simulink model "matlab_mixed_cosim"  (Simulink 7.0)
settings: Solver=FixedStepDiscrete  SolverMode=SingleTasking  StartTime=0.0  StopTime=370  RelTol=1e-3
undefined symbols (not defined in the file or in its folder): ieee_nowarn, image, port_label
libraries: aldec_ahdl x7
settings Model: Creator=arekg  LastModifiedBy=arekg
settings DataIOCC: SignalLoggingName=sigsOut
settings OptimizationCC: InlineInvariantSignals=on
settings DebuggingCC: SaveWithParameterizedLinksMsg=none  SignalResolutionControl=TryResolveAllWithWarning  SolverPrmCheckMsg=none  MultiTaskDSMMsg=warning  MultiTaskCondExecSysMsg=none
settings HardwareCC: TargetUnknown=on
settings RTWCC: IncludeERTFirstTime=on
settings GRTTargetCC: TargetFcnLib=ansi_tfl_tmw.mat  ModelReferenceCompliant=off  MatFileLogging=off

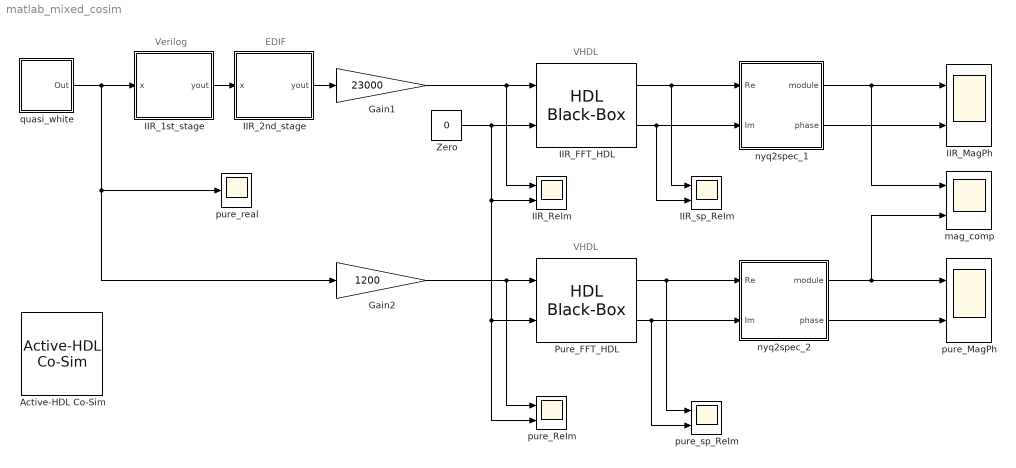
== system matlab_mixed_cosim ==
  note: Verilog
  note: EDIF
  note: VHDL
  note: VHDL
  Active-HDL Co-Sim : aldec_ahdl/Active-HDL Co-Sim  Tag=Active-HDL_Co-Sim_close  Priority=1  hdl_period=0.5  hdl_tscale=sec  sys_period=[1, 0]  sys_tscale=As In Simulator  vsim_cmd=-ieee_nowarn  wav_fn=matlab_mixed_cosim  wav_settings=[0,0,0,0,0,0,0,0]  dbg=off  auto_start=off  gen_tb=[0,0,0]  batch_sim=off  tb_fn=mlab_post_tb.log  metavalue_map=[0,0]  sim_resolution=[1,0,0]  active_page=4  aws_en=off  ahdl_en=off  blk_ver=9.3.RTM  macro_en=[1,0,1]  macro_path=prepare_project.do  mfun_text=check_mfiles
  Gain1 : Gain  Gain=23000  ParameterDataType=sfix(16)  ParameterScaling=2^0  OutDataType=sfix(16)  OutScaling=2^0  SaturateOnIntegerOverflow=on
  Gain2 : Gain  Gain=1200  ParameterDataType=sfix(16)  ParameterScaling=2^0  OutDataType=sfix(16)  OutScaling=2^0  SaturateOnIntegerOverflow=on
  IIR_1st_stage : Subsystem
  IIR_2nd_stage : Subsystem
  IIR_FFT_HDL : aldec_ahdl/HDL Black-Box  Priority=1  module_m=top_fft  ports_cfg={ce,4,1,0,0,1,8,0,0,1,0,0}{clk,3,1,0,0,1,8,0,0,1,0,0}{inv,5,1,0,0,1,8,0,0,1,0,0}{rst,5,1,0,0,1,8,0,0,1,0,0}{start,5,1,0,0,1,8,0,0,1,0,0}{Iin,0,-1,0,0,Inherited,0,0,0,0,0,0}{Qin,0,-1,0,0,Inherited,0,0,0,0,0,0}{Iout,1,-1,0,0,clk,0,0,0,0,0,0}{Qout,1,-1,0,0,clk,0,0,0,0,0,0}  params={WIDTH,16,NATURAL}{POINT,64,NATURAL}{STAGE,3,NATURAL}  clocks={1,2,0,0.5000,0}  ces={0,1,1,0,1}  stims={3,1 0s 0 7s}{4,0 0s 1 8s 0 10s}{2,0}  hdl_src=c:\My_Designs\Samples_73\simulink_mixed_example\fft\src\cfft\address.vhd;c:\My_Designs\Samples_73\simulink_mixed_example\fft\src\cfft\blockdram.vhd;c:\My_Designs\Samples_73\simulink_mixed_example\fft\src\cfft\div4limit.vhd;c:\My_Designs\Samples_73\simulink_mixed_example\fft\src\cfft\cfft4.vhd;c:\My_Designs\Samples_73\simulink_mixed_example\fft\src\cfft\rofactor.vhd;c:\My_Designs\Samples_73\simulink_mixed_example\fft\src\cfft\p2r_cordic.vhd;c:\My_Designs\Samples_73\simulink_mixed_example\fft\src\cfft\sc_corproc.vhd;c:\My_Designs\Samples_73\simulink_mixed_example\fft\src\cfft\mulfactor.vhd;c:\My_Designs\Samples_73\simulink_mixed_example\fft\src\cfft\cfft.vhd;c:\My_Designs\Samples_73\simulink_mixed_example\fft\src\ram\ram.vhd;c:\My_Designs\Samples_73\simulink_mixed_example\fft\compile\control.vhd;c:\My_Designs\Samples_73\simulink_mixed_example\fft\compile\top_fft.vhd  block_mask=image(imread('HDLBlackBox.jpg'),'center'); disp('top_fft');port_label('input', 1, 'Iin');port_label('input', 2, 'Qin');port_label('output', 1, 'Iout');port_label('output', 2, 'Qout');  config=[2,2]  inp=[2, 0, abs(16-1 - 0) + 1, 0, 0, 0, 0, 0, abs(16-1 - 0) + 1, 0, 0, 0, 0]  out=[2, 0, abs(16+1 - 0) + 1, 0, 0, 0, 0, 0, abs(16+1 - 0) + 1, 0, 0, 0, 0]  sampling=[1,-1,-1,2,2]  active_page={0}{80,0,35,1,65,2,70,3,70,4,60,5,60,6,50,7,35,8,35,9,119,10}{103,0,55,1,70,2,75,3,75,4,45,5,45,6,45,7,165,8,0,0,0,0}{165,0,130,1,190,2,190,3,0,0,0,0,0,0,0,0,0,0,0,0,0,0}{81,0,60,1,60,2,70,3,60,4,0,0,0,0,0,0,0,0,0,0,0,0}{83,0,70,1,80,2,50,3,50,4,0,0,0,0,0,0,0,0,0,0,0,0}{125,0,330,1,220,2,0,0,0,0,0,0,0,0,0,0,0,0,0,0,0,0}{95,0,95,1,70,2,50,3,80,4,35,5,35,6,65,7,150,8,0,0,0,0}{735,436}  param_val={16,-1,64,-1,3,-1}  clk_val=[2,0,0.5000]  ce_val=[1,0]  blk_ver=9.3.RTM  blk_conf=0  user_conv=0
  IIR_MagPh : Scope  NumInputPorts=2
      settings: YMin=0~-2  YMax=11500~3.25
  IIR_ReIm : Scope  NumInputPorts=2
      settings: YMin=-25000~-1  YMax=25000~1  SaveName=ScopeData19
  IIR_sp_ReIm : Scope  NumInputPorts=2
      settings: YMin=-35000~-35000  YMax=35000~35000  SaveName=ScopeData5
  Pure_FFT_HDL : aldec_ahdl/HDL Black-Box  Priority=1  module_m=top_fft  ports_cfg={ce,4,1,0,0,1,8,0,0,1,0,0}{clk,3,1,0,0,1,8,0,0,1,0,0}{inv,5,1,0,0,1,8,0,0,1,0,0}{rst,5,1,0,0,1,8,0,0,1,0,0}{start,5,1,0,0,1,8,0,0,1,0,0}{Iin,0,-1,0,0,Inherited,0,0,0,0,0,0}{Qin,0,-1,0,0,Inherited,0,0,0,0,0,0}{Iout,1,-1,0,0,clk,0,0,0,0,0,0}{Qout,1,-1,0,0,clk,0,0,0,0,0,0}  params={WIDTH,16,NATURAL}{POINT,64,NATURAL}{STAGE,3,NATURAL}  clocks={1,2,0,0.5000,0}  ces={0,1,1,0,1}  stims={3,1 0s 0 7s}{4,0 0s 1 8s 0 10s}{2,0}  hdl_src=c:\My_Designs\Samples_73\simulink_mixed_example\fft\src\cfft\address.vhd;c:\My_Designs\Samples_73\simulink_mixed_example\fft\src\cfft\blockdram.vhd;c:\My_Designs\Samples_73\simulink_mixed_example\fft\src\cfft\div4limit.vhd;c:\My_Designs\Samples_73\simulink_mixed_example\fft\src\cfft\cfft4.vhd;c:\My_Designs\Samples_73\simulink_mixed_example\fft\src\cfft\rofactor.vhd;c:\My_Designs\Samples_73\simulink_mixed_example\fft\src\cfft\p2r_cordic.vhd;c:\My_Designs\Samples_73\simulink_mixed_example\fft\src\cfft\sc_corproc.vhd;c:\My_Designs\Samples_73\simulink_mixed_example\fft\src\cfft\mulfactor.vhd;c:\My_Designs\Samples_73\simulink_mixed_example\fft\src\cfft\cfft.vhd;c:\My_Designs\Samples_73\simulink_mixed_example\fft\src\ram\ram.vhd;c:\My_Designs\Samples_73\simulink_mixed_example\fft\compile\control.vhd;c:\My_Designs\Samples_73\simulink_mixed_example\fft\compile\top_fft.vhd  block_mask=image(imread('HDLBlackBox.jpg'),'center'); disp('top_fft');port_label('input', 1, 'Iin');port_label('input', 2, 'Qin');port_label('output', 1, 'Iout');port_label('output', 2, 'Qout');  config=[2,2]  inp=[2, 0, abs(16-1 - 0) + 1, 0, 0, 0, 0, 0, abs(16-1 - 0) + 1, 0, 0, 0, 0]  out=[2, 0, abs(16+1 - 0) + 1, 0, 0, 0, 0, 0, abs(16+1 - 0) + 1, 0, 0, 0, 0]  sampling=[1,-1,-1,2,2]  active_page={0}{80,0,35,1,65,2,70,3,70,4,60,5,60,6,50,7,35,8,35,9,119,10}{103,0,55,1,70,2,75,3,75,4,45,5,45,6,45,7,165,8,0,0,0,0}{165,0,130,1,190,2,190,3,0,0,0,0,0,0,0,0,0,0,0,0,0,0}{81,0,60,1,60,2,70,3,60,4,0,0,0,0,0,0,0,0,0,0,0,0}{83,0,70,1,80,2,50,3,50,4,0,0,0,0,0,0,0,0,0,0,0,0}{125,0,330,1,220,2,0,0,0,0,0,0,0,0,0,0,0,0,0,0,0,0}{95,0,95,1,70,2,50,3,80,4,35,5,35,6,65,7,150,8,0,0,0,0}{735,436}  param_val={16,-1,64,-1,3,-1}  clk_val=[2,0,0.5000]  ce_val=[1,0]  blk_ver=9.3.RTM  blk_conf=0  user_conv=0
  Zero : Constant  Value=0  OutDataTypeMode=double  OutDataType=sfix(16)  OutScaling=2^0
  mag_comp : Scope  NumInputPorts=2
      settings: TimeRange=370  YMin=0~0  YMax=12000~7000
  nyq2spec_1 : Subsystem
  nyq2spec_2 : Subsystem
  pure_MagPh : Scope  NumInputPorts=2
      settings: TimeRange=370  YMin=-3.5~-5  YMax=3.5~5  SaveName=ScopeData24
  pure_ReIm : Scope  NumInputPorts=2
      settings: YMin=-1200~-1  YMax=1200~1  SaveName=ScopeData21
  pure_real : Scope
      settings: YMin=-450  YMax=450  SaveName=ScopeData13
  pure_sp_ReIm : Scope  NumInputPorts=2
      settings: YMin=-1~-5  YMax=1~5  SaveName=ScopeData20
  quasi_white : Subsystem
  wires:
  IIR_FFT_HDL/1 -> IIR_sp_ReIm/1, nyq2spec_1/1(Re)
  IIR_FFT_HDL/2 -> IIR_sp_ReIm/2, nyq2spec_1/2(Im)
  nyq2spec_1/1(module) -> IIR_MagPh/1, mag_comp/1
  nyq2spec_1/2(phase) -> IIR_MagPh/2
  Zero/1 -> IIR_FFT_HDL/2, IIR_ReIm/2, pure_ReIm/2, Pure_FFT_HDL/2
  quasi_white/1(Out) -> pure_real/1, IIR_1st_stage/1(x), Gain2/1
  nyq2spec_2/1(module) -> pure_MagPh/1, mag_comp/2
  Gain1/1 -> IIR_ReIm/1, IIR_FFT_HDL/1
  IIR_1st_stage/1(yout) -> IIR_2nd_stage/1(x)
  Pure_FFT_HDL/1 -> nyq2spec_2/1(Re), pure_sp_ReIm/1
  Gain2/1 -> pure_ReIm/1, Pure_FFT_HDL/1
  Pure_FFT_HDL/2 -> nyq2spec_2/2(Im), pure_sp_ReIm/2
  nyq2spec_2/2(phase) -> pure_MagPh/2
  IIR_2nd_stage/1(yout) -> Gain1/1

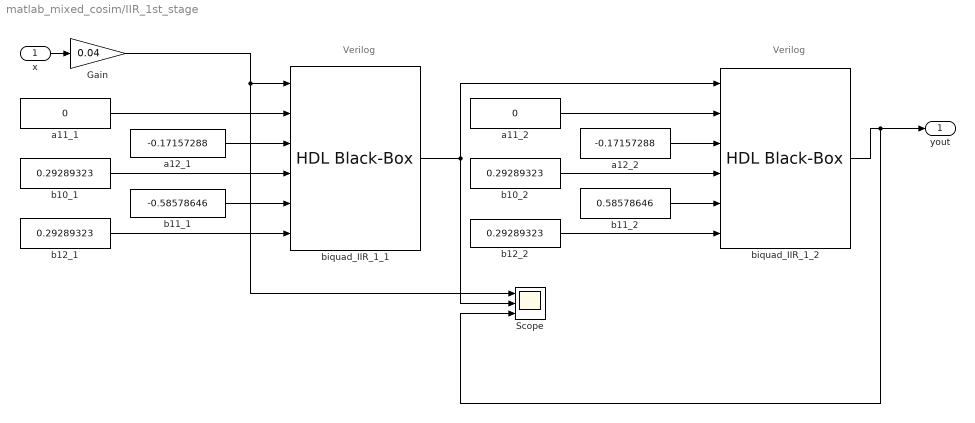
== system matlab_mixed_cosim/IIR_1st_stage ==
  note: Verilog
  note: Verilog
  x : Inport  OutDataType=sfix(16)  OutScaling=2^0
  Gain : Gain  Gain=0.04  ParameterDataType=sfix(16)  ParameterScaling=2^0  OutDataType=sfix(16)  OutScaling=2^0  SaturateOnIntegerOverflow=on
  Scope : Scope  NumInputPorts=3
      settings: YMin=-0.025~-0.025~-0.02  YMax=0.025~0.03~0.03  SaveName=ScopeData3
  a11_1 : Constant  Value=0  OutDataType=sfix(16)  OutScaling=2^0
  a11_2 : Constant  Value=0  OutDataType=sfix(16)  OutScaling=2^0
  a12_1 : Constant  Value=-0.17157288  OutDataType=sfix(16)  OutScaling=2^0
  a12_2 : Constant  Value=-0.17157288  OutDataType=sfix(16)  OutScaling=2^0
  b10_1 : Constant  Value=0.29289323  OutDataType=sfix(16)  OutScaling=2^0
  b10_2 : Constant  Value=0.29289323  OutDataType=sfix(16)  OutScaling=2^0
  b11_1 : Constant  Value=-0.58578646  OutDataType=sfix(16)  OutScaling=2^0
  b11_2 : Constant  Value=0.58578646  OutDataType=sfix(16)  OutScaling=2^0
  b12_1 : Constant  Value=0.29289323  OutDataType=sfix(16)  OutScaling=2^0
  b12_2 : Constant  Value=0.29289323  OutDataType=sfix(16)  OutScaling=2^0
  biquad_IIR_1_1 : aldec_ahdl/HDL Black-Box  Priority=1  module_m=biquad  ports_cfg={clk,3,1,0,0,1,8,0,0,1,0,0}{nreset,5,1,0,0,1,8,0,0,1,0,0}{x,0,16,0,15,Inherited,0,0,0,0,0,0}{ce,4,1,0,0,1,8,0,0,1,0,0}{valid,5,1,0,0,1,8,0,0,1,0,0}{a11,0,8,0,7,Inherited,0,0,0,0,0,0}{a12,0,8,0,7,Inherited,0,0,0,0,0,0}{b10,0,8,0,7,Inherited,0,0,0,0,0,0}{b11,0,8,0,7,Inherited,0,0,0,0,0,0}{b12,0,8,0,7,Inherited,0,0,0,0,0,0}{yout,1,16,0,15,clk,0,0,0,0,0,0}  params={DATAWIDTH,16,}{COEFWIDTH,8,}{ACCUM,2,}  clocks={0,2,0,0.5000,0}  ces={3,0,1,0,1}  stims={4,0 0s 1 2s}{1,0 0s 1 2s}  hdl_src=c:\My_Designs\Samples_73\simulink_mixed_example\biquad_iir\src\multa.v;c:\My_Designs\Samples_73\simulink_mixed_example\biquad_iir\src\multb.v;c:\My_Designs\Samples_73\simulink_mixed_example\biquad_iir\src\biquad.v  block_mask=image(imread('HDLBlackBox.jpg'),'center'); disp('biquad');port_label('input', 1, 'x');port_label('input', 2, 'a11');port_label('input', 3, 'a12');port_label('input', 4, 'b10');port_label('input', 5, 'b11');port_label('input', 6, 'b12');port_label('output', 1, 'yout');  config=[6,1]  inp=[6, 0, 16, 15, 0, 0, 0, 0, 8, 7, 0, 0, 0, 0, 8, 7, 0, 0, 0, 0, 8, 7, 0, 0, 0, 0, 8, 7, 0, 0, 0, 0, 8, 7, 0, 0, 0]  out=[1, 0, 16, 15, 0, 0, 0]  sampling=[1,-1,-1,-1,-1,-1,-1,2]  active_page={0}{80,0,35,1,65,2,70,3,70,4,60,5,60,6,50,7,35,8,35,9,119,10}{103,0,55,1,70,2,75,3,75,4,45,5,45,6,45,7,165,8,0,0,0,0}{165,0,130,1,190,2,190,3,0,0,0,0,0,0,0,0,0,0,0,0,0,0}{81,0,60,1,60,2,70,3,60,4,0,0,0,0,0,0,0,0,0,0,0,0}{83,0,70,1,80,2,50,3,50,4,0,0,0,0,0,0,0,0,0,0,0,0}{125,0,330,1,220,2,0,0,0,0,0,0,0,0,0,0,0,0,0,0,0,0}{95,0,95,1,70,2,50,3,80,4,35,5,35,6,65,7,150,8,0,0,0,0}{735,436}  param_val={16,-1,8,-1,2,-1}  clk_val=[2,0,0.5000]  ce_val=[1,0]  blk_ver=9.3.RTM  blk_conf=0  user_conv=0
  biquad_IIR_1_2 : aldec_ahdl/HDL Black-Box  Priority=1  module_m=biquad  ports_cfg={clk,3,1,0,0,1,8,0,0,1,0,0}{nreset,5,1,0,0,1,8,0,0,1,0,0}{x,0,16,0,15,Inherited,0,0,0,0,0,0}{ce,4,1,0,0,1,8,0,0,1,0,0}{valid,5,1,0,0,1,8,0,0,1,0,0}{a11,0,8,0,7,Inherited,0,0,0,0,0,0}{a12,0,8,0,7,Inherited,0,0,0,0,0,0}{b10,0,8,0,7,Inherited,0,0,0,0,0,0}{b11,0,8,0,7,Inherited,0,0,0,0,0,0}{b12,0,8,0,7,Inherited,0,0,0,0,0,0}{yout,1,16,0,15,clk,0,0,0,0,0,0}  params={DATAWIDTH,16,}{COEFWIDTH,8,}{ACCUM,2,}  clocks={0,2,0,0.5000,0}  ces={3,0,1,0,1}  stims={4,0 0s 1 2s}{1,0 0s 1 2s}  hdl_src=c:\My_Designs\Samples_73\simulink_mixed_example\biquad_iir\src\multa.v;c:\My_Designs\Samples_73\simulink_mixed_example\biquad_iir\src\multb.v;c:\My_Designs\Samples_73\simulink_mixed_example\biquad_iir\src\biquad.v  block_mask=image(imread('HDLBlackBox.jpg'),'center'); disp('biquad');port_label('input', 1, 'x');port_label('input', 2, 'a11');port_label('input', 3, 'a12');port_label('input', 4, 'b10');port_label('input', 5, 'b11');port_label('input', 6, 'b12');port_label('output', 1, 'yout');  config=[6,1]  inp=[6, 0, 16, 15, 0, 0, 0, 0, 8, 7, 0, 0, 0, 0, 8, 7, 0, 0, 0, 0, 8, 7, 0, 0, 0, 0, 8, 7, 0, 0, 0, 0, 8, 7, 0, 0, 0]  out=[1, 0, 16, 15, 0, 0, 0]  sampling=[1,-1,-1,-1,-1,-1,-1,2]  active_page={0}{80,0,35,1,65,2,70,3,70,4,60,5,60,6,50,7,35,8,35,9,119,10}{103,0,55,1,70,2,75,3,75,4,45,5,45,6,45,7,165,8,0,0,0,0}{165,0,130,1,190,2,190,3,0,0,0,0,0,0,0,0,0,0,0,0,0,0}{81,0,60,1,60,2,70,3,60,4,0,0,0,0,0,0,0,0,0,0,0,0}{83,0,70,1,80,2,50,3,50,4,0,0,0,0,0,0,0,0,0,0,0,0}{125,0,330,1,220,2,0,0,0,0,0,0,0,0,0,0,0,0,0,0,0,0}{95,0,95,1,70,2,50,3,80,4,35,5,35,6,65,7,150,8,0,0,0,0}{735,436}  param_val={16,-1,8,-1,2,-1}  clk_val=[2,0,0.5000]  ce_val=[1,0]  blk_ver=9.3.RTM  blk_conf=0  user_conv=0
  yout : Outport  OutDataType=sfix(16)  OutScaling=2^0
  wires:
  x/1 -> Gain/1
  biquad_IIR_1_1/1 -> biquad_IIR_1_2/1, Scope/2
  Gain/1 -> biquad_IIR_1_1/1, Scope/1
  biquad_IIR_1_2/1 -> yout/1, Scope/3
  b10_1/1 -> biquad_IIR_1_1/4
  a12_1/1 -> biquad_IIR_1_1/3
  a11_1/1 -> biquad_IIR_1_1/2
  b12_2/1 -> biquad_IIR_1_2/6
  b10_2/1 -> biquad_IIR_1_2/4
  a12_2/1 -> biquad_IIR_1_2/3
  a11_2/1 -> biquad_IIR_1_2/2
  b11_2/1 -> biquad_IIR_1_2/5
  b12_1/1 -> biquad_IIR_1_1/6
  b11_1/1 -> biquad_IIR_1_1/5

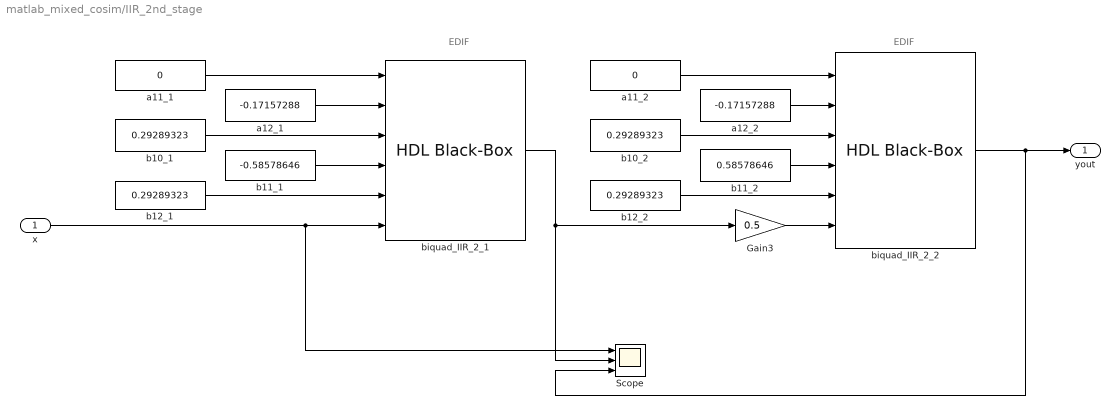
== system matlab_mixed_cosim/IIR_2nd_stage ==
  note: EDIF
  note: EDIF
  x : Inport  OutDataType=sfix(16)  OutScaling=2^0
  Gain3 : Gain  Gain=0.5  ParameterDataType=sfix(16)  ParameterScaling=2^0  OutDataType=sfix(16)  OutScaling=2^0  SaturateOnIntegerOverflow=on
  Scope : Scope  NumInputPorts=3
      settings: YMin=-0.025~-0.025~-0.02  YMax=0.025~0.03~0.03  SaveName=ScopeData4
  a11_1 : Constant  Value=0  OutDataType=sfix(16)  OutScaling=2^0
  a11_2 : Constant  Value=0  OutDataType=sfix(16)  OutScaling=2^0
  a12_1 : Constant  Value=-0.17157288  OutDataType=sfix(16)  OutScaling=2^0
  a12_2 : Constant  Value=-0.17157288  OutDataType=sfix(16)  OutScaling=2^0
  b10_1 : Constant  Value=0.29289323  OutDataType=sfix(16)  OutScaling=2^0
  b10_2 : Constant  Value=0.29289323  OutDataType=sfix(16)  OutScaling=2^0
  b11_1 : Constant  Value=-0.58578646  OutDataType=sfix(16)  OutScaling=2^0
  b11_2 : Constant  Value=0.58578646  OutDataType=sfix(16)  OutScaling=2^0
  b12_1 : Constant  Value=0.29289323  OutDataType=sfix(16)  OutScaling=2^0
  b12_2 : Constant  Value=0.29289323  OutDataType=sfix(16)  OutScaling=2^0
  biquad_IIR_2_1 : aldec_ahdl/HDL Black-Box  Priority=1  module_m=biquad_post_synth  ports_cfg={a11,0,8,0,7,Inherited,0,0,0,0,0,0}{a12,0,8,0,7,Inherited,0,0,0,0,0,0}{b10,0,8,0,7,Inherited,0,0,0,0,0,0}{b11,0,8,0,7,Inherited,0,0,0,0,0,0}{b12,0,8,0,7,Inherited,0,0,0,0,0,0}{x,0,16,0,15,Inherited,0,0,0,0,0,0}{ce,4,1,0,0,1,8,0,0,1,0,0}{clk,3,1,0,0,1,8,0,0,1,0,0}{nreset,5,1,0,0,1,8,0,0,1,0,0}{valid,5,1,0,0,1,8,0,0,1,0,0}{yout,1,16,0,15,clk,0,0,0,0,0,0}  clocks={7,2,0,0.5000,0}  ces={6,7,1,0,1}  stims={8,0 0s 1 2s}{9,0 0s 1 2s}  hdl_src=C:\Program Files\Aldec\Active-HDL 7.2\Vlib\VIRTEX\src\virtex.vhd;C:\Program Files\Aldec\Active-HDL 7.2\Vlib\unisim\src\unisim_vital.vhd;c:\My_Designs\Samples_73\simulink_mixed_example\biquad_iir\src\post-synthesis\biquad_post_synth.edf  block_mask=image(imread('HDLBlackBox.jpg'),'center'); disp('biquad_post_synth');port_label('input', 1, 'a11');port_label('input', 2, 'a12');port_label('input', 3, 'b10');port_label('input', 4, 'b11');port_label('input', 5, 'b12');port_label('input', 6, 'x');port_label('output', 1, 'yout');  config=[6,1]  inp=[6, 0, 8, 7, 0, 0, 0, 0, 8, 7, 0, 0, 0, 0, 8, 7, 0, 0, 0, 0, 8, 7, 0, 0, 0, 0, 8, 7, 0, 0, 0, 0, 16, 15, 0, 0, 0]  out=[1, 0, 16, 15, 0, 0, 0]  sampling=[1,-1,-1,-1,-1,-1,-1,2]  active_page={0}{80,0,35,1,65,2,70,3,70,4,60,5,60,6,50,7,35,8,35,9,119,10}{103,0,55,1,70,2,75,3,75,4,45,5,45,6,45,7,165,8,0,0,0,0}{165,0,130,1,190,2,190,3,0,0,0,0,0,0,0,0,0,0,0,0,0,0}{81,0,60,1,60,2,70,3,60,4,0,0,0,0,0,0,0,0,0,0,0,0}{83,0,70,1,80,2,50,3,50,4,0,0,0,0,0,0,0,0,0,0,0,0}{125,0,330,1,220,2,0,0,0,0,0,0,0,0,0,0,0,0,0,0,0,0}{95,0,95,1,70,2,50,3,80,4,35,5,35,6,65,7,150,8,0,0,0,0}{735,436}  param_val=0  clk_val=[2,0,0.5000]  ce_val=[1,0]  blk_ver=9.3.RTM  blk_conf=0  user_conv=0
  biquad_IIR_2_2 : aldec_ahdl/HDL Black-Box  Priority=1  module_m=biquad_post_synth  ports_cfg={a11,0,8,0,7,Inherited,0,0,0,0,0,0}{a12,0,8,0,7,Inherited,0,0,0,0,0,0}{b10,0,8,0,7,Inherited,0,0,0,0,0,0}{b11,0,8,0,7,Inherited,0,0,0,0,0,0}{b12,0,8,0,7,Inherited,0,0,0,0,0,0}{x,0,16,0,15,Inherited,0,0,0,0,0,0}{ce,4,1,0,0,1,8,0,0,1,0,0}{clk,3,1,0,0,1,8,0,0,1,0,0}{nreset,5,1,0,0,1,8,0,0,1,0,0}{valid,5,1,0,0,1,8,0,0,1,0,0}{yout,1,16,0,15,clk,0,0,0,0,0,0}  clocks={7,2,0,0.5000,0}  ces={6,7,1,0,1}  stims={8,0 0s 1 2s}{9,0 0s 1 2s}  hdl_src=C:\Program Files\Aldec\Active-HDL 7.2\Vlib\VIRTEX\src\virtex.vhd;C:\Program Files\Aldec\Active-HDL 7.2\Vlib\unisim\src\unisim_vital.vhd;c:\My_Designs\Samples_73\simulink_mixed_example\biquad_iir\src\post-synthesis\biquad_post_synth.edf  block_mask=image(imread('HDLBlackBox.jpg'),'center'); disp('biquad_post_synth');port_label('input', 1, 'a11');port_label('input', 2, 'a12');port_label('input', 3, 'b10');port_label('input', 4, 'b11');port_label('input', 5, 'b12');port_label('input', 6, 'x');port_label('output', 1, 'yout');  config=[6,1]  inp=[6, 0, 8, 7, 0, 0, 0, 0, 8, 7, 0, 0, 0, 0, 8, 7, 0, 0, 0, 0, 8, 7, 0, 0, 0, 0, 8, 7, 0, 0, 0, 0, 16, 15, 0, 0, 0]  out=[1, 0, 16, 15, 0, 0, 0]  sampling=[1,-1,-1,-1,-1,-1,-1,2]  active_page={0}{80,0,35,1,65,2,70,3,70,4,60,5,60,6,50,7,35,8,35,9,119,10}{103,0,55,1,70,2,75,3,75,4,45,5,45,6,45,7,165,8,0,0,0,0}{165,0,130,1,190,2,190,3,0,0,0,0,0,0,0,0,0,0,0,0,0,0}{81,0,60,1,60,2,70,3,60,4,0,0,0,0,0,0,0,0,0,0,0,0}{83,0,70,1,80,2,50,3,50,4,0,0,0,0,0,0,0,0,0,0,0,0}{125,0,330,1,220,2,0,0,0,0,0,0,0,0,0,0,0,0,0,0,0,0}{95,0,95,1,70,2,50,3,80,4,35,5,35,6,65,7,150,8,0,0,0,0}{735,436}  param_val=0  clk_val=[2,0,0.5000]  ce_val=[1,0]  blk_ver=9.3.RTM  blk_conf=0  user_conv=0
  yout : Outport  OutDataType=sfix(16)  OutScaling=2^0
  wires:
  biquad_IIR_2_1/1 -> Scope/2, Gain3/1
  biquad_IIR_2_2/1 -> Scope/3, yout/1
  b10_1/1 -> biquad_IIR_2_1/3
  a12_1/1 -> biquad_IIR_2_1/2
  a11_1/1 -> biquad_IIR_2_1/1
  b12_2/1 -> biquad_IIR_2_2/5
  b10_2/1 -> biquad_IIR_2_2/3
  a12_2/1 -> biquad_IIR_2_2/2
  a11_2/1 -> biquad_IIR_2_2/1
  b11_2/1 -> biquad_IIR_2_2/4
  b12_1/1 -> biquad_IIR_2_1/5
  b11_1/1 -> biquad_IIR_2_1/4
  Gain3/1 -> biquad_IIR_2_2/6
  x/1 -> Scope/1, biquad_IIR_2_1/6

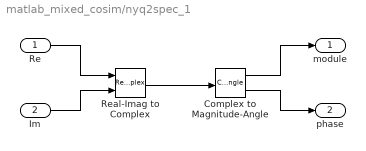
== system matlab_mixed_cosim/nyq2spec_1 ==
  Re : Inport  OutDataType=sfix(16)  OutScaling=2^0
  Im : Inport  Port=2  OutDataType=sfix(16)  OutScaling=2^0
  Complex to Magnitude-Angle : ComplexToMagnitudeAngle
  Real-Imag to Complex : RealImagToComplex
  module : Outport  OutDataType=sfix(16)  OutScaling=2^0
  phase : Outport  Port=2  OutDataType=sfix(16)  OutScaling=2^0
  wires:
  Re/1 -> Real-Imag to Complex/1
  Real-Imag to Complex/1 -> Complex to Magnitude-Angle/1
  Complex to Magnitude-Angle/1 -> module/1
  Im/1 -> Real-Imag to Complex/2
  Complex to Magnitude-Angle/2 -> phase/1

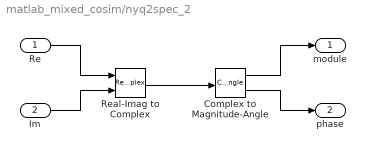
== system matlab_mixed_cosim/nyq2spec_2 ==
  Re : Inport  OutDataType=sfix(16)  OutScaling=2^0
  Im : Inport  Port=2  OutDataType=sfix(16)  OutScaling=2^0
  Complex to Magnitude-Angle : ComplexToMagnitudeAngle
  Real-Imag to Complex : RealImagToComplex
  module : Outport  OutDataType=sfix(16)  OutScaling=2^0
  phase : Outport  Port=2  OutDataType=sfix(16)  OutScaling=2^0
  wires:
  Re/1 -> Real-Imag to Complex/1
  Real-Imag to Complex/1 -> Complex to Magnitude-Angle/1
  Complex to Magnitude-Angle/1 -> module/1
  Im/1 -> Real-Imag to Complex/2
  Complex to Magnitude-Angle/2 -> phase/1

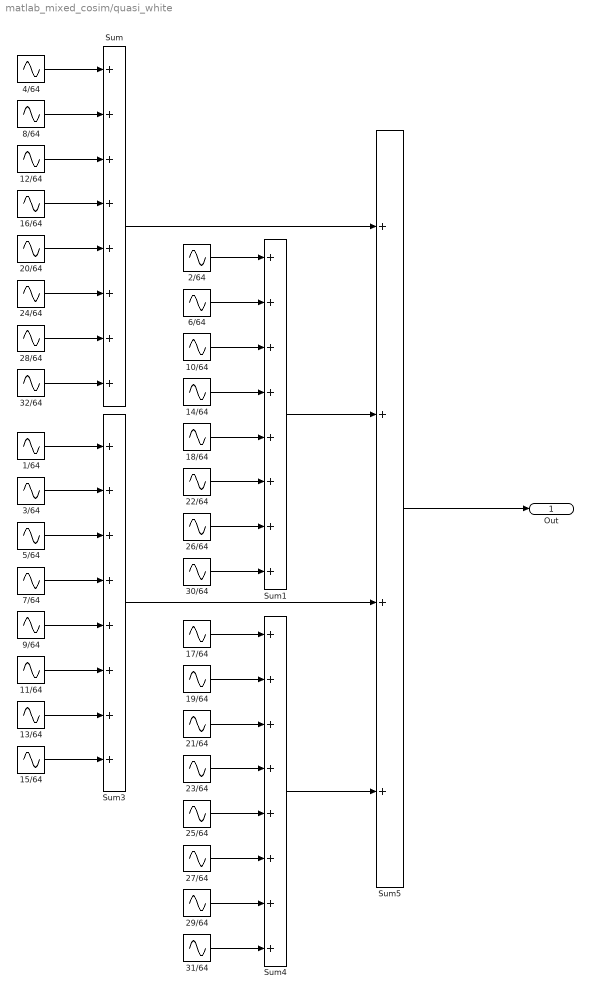
== system matlab_mixed_cosim/quasi_white ==
  1/64 : Sin  Frequency=0.09817  Samples=0.0625  SampleTime=1
  10/64 : Sin  Frequency=0.98175  Samples=4  SampleTime=1
  11/64 : Sin  Frequency=1.07992  Samples=4  SampleTime=1
  12/64 : Sin  Frequency=1.1781  Samples=4  SampleTime=1
  13/64 : Sin  Frequency=1.27627  Samples=4  SampleTime=1
  14/64 : Sin  Frequency=1.37445  Samples=6  SampleTime=1
  15/64 : Sin  Frequency=1.47262  Samples=0.0625  SampleTime=1
  16/64 : Sin  Frequency=1.5708  Samples=6  SampleTime=1
  17/64 : Sin  Frequency=1.66897  Samples=0.125  SampleTime=1
  18/64 : Sin  Frequency=1.76715  Samples=0.3125  SampleTime=1
  19/64 : Sin  Frequency=1.86532  Samples=4  SampleTime=1
  2/64 : Sin  Frequency=0.19635  Samples=0.0625  SampleTime=1
  20/64 : Sin  Frequency=1.9635  Samples=0.3125  SampleTime=1
  21/64 : Sin  Frequency=2.06167  Samples=6  SampleTime=1
  22/64 : Sin  Frequency=2.15984  Samples=4  SampleTime=1
  23/64 : Sin  Frequency=2.25802  Samples=0.3125  SampleTime=1
  24/64 : Sin  Frequency=2.3562  Samples=4  SampleTime=1
  25/64 : Sin  Frequency=2.45437  Samples=4  SampleTime=1
  26/64 : Sin  Frequency=2.55254  Samples=4  SampleTime=1
  27/64 : Sin  Frequency=2.65072  Samples=4  SampleTime=1
  28/64 : Sin  Frequency=2.74889  Samples=4  SampleTime=1
  "29/64 " : Sin  Frequency=2.84707  Samples=4  SampleTime=1
  3/64 : Sin  Frequency=0.29452  Samples=0.125  SampleTime=1
  30/64 : Sin  Frequency=2.94524  Samples=4  SampleTime=1
  31/64 : Sin  Frequency=3.04342  Samples=4  SampleTime=1
  32/64 : Sin  Frequency=3.14159  Samples=4  SampleTime=1
  4/64 : Sin  Frequency=0.3927  Samples=0.0625  SampleTime=1
  5/64 : Sin  Frequency=0.49087  Samples=4  SampleTime=1
  6/64 : Sin  Frequency=0.58905  Samples=0.125  SampleTime=1
  7/64 : Sin  Frequency=0.68722  Samples=6  SampleTime=1
  8/64 : Sin  Frequency=0.7854  Samples=0.125  SampleTime=1
  9/64 : Sin  Frequency=0.88357  Samples=0.3125  SampleTime=1
  Sum{,1,3..4} (4 alike) : Sum  Inputs=++++++++  OutDataType=sfix(16)  OutScaling=2^0  SaturateOnIntegerOverflow=on
  Sum5 : Sum  Inputs=++++  OutDataType=sfix(16)  OutScaling=2^0  SaturateOnIntegerOverflow=on
  Out : Outport  OutDataType=sfix(16)  OutScaling=2^0
  wires:
  24/64/1 -> Sum/6
  20/64/1 -> Sum/5
  16/64/1 -> Sum/4
  12/64/1 -> Sum/3
  8/64/1 -> Sum/2
  4/64/1 -> Sum/1
  22/64/1 -> Sum1/6
  18/64/1 -> Sum1/5
  14/64/1 -> Sum1/4
  10/64/1 -> Sum1/3
  6/64/1 -> Sum1/2
  2/64/1 -> Sum1/1
  Sum/1 -> Sum5/1
  28/64/1 -> Sum/7
  26/64/1 -> Sum1/7
  11/64/1 -> Sum3/6
  9/64/1 -> Sum3/5
  7/64/1 -> Sum3/4
  5/64/1 -> Sum3/3
  3/64/1 -> Sum3/2
  Sum3/1 -> Sum5/3
  13/64/1 -> Sum3/7
  1/64/1 -> Sum3/1
  Sum1/1 -> Sum5/2
  Sum4/1 -> Sum5/4
  32/64/1 -> Sum/8
  30/64/1 -> Sum1/8
  15/64/1 -> Sum3/8
  25/64/1 -> Sum4/5
  23/64/1 -> Sum4/4
  21/64/1 -> Sum4/3
  19/64/1 -> Sum4/2
  17/64/1 -> Sum4/1
  27/64/1 -> Sum4/6
  "29/64 "/1 -> Sum4/7
  31/64/1 -> Sum4/8
  Sum5/1 -> Out/1
